simulink model "mdl"  (R2022b)
settings: Solver=VariableStepAuto  StartTime=0.0  StopTime=10.0  RelTol=1e-3
values from neighbouring files (symbols this model uses):
  acc_g = 9.8    [load_init_states.m]
  CG = [0;0;0]    [load_init_states.m]
  CP = [0;0;0]    [load_mdl_data.m]
  h0 = 1    [load_init_states.m]
  mass = 38    [load_init_states.m]
  maxP = 3000*0.8    (= 2400)    [load_mdl_data.m]
libraries: aerospace_common x3, aero x1, aerolibatmos2 x1
settings Model: Creator=matt  LastModifiedBy=matt
settings DataIOCC: ExternalInput=getinputstruct(spec1)  InitialState=getstatestruct(spec1)

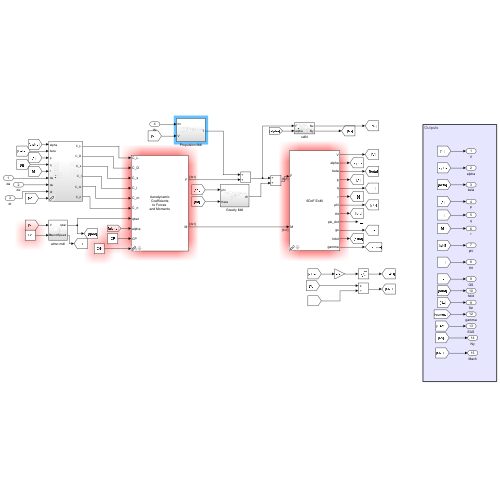
[thumbnail: Simulink's stored preview of the top-level diagram]
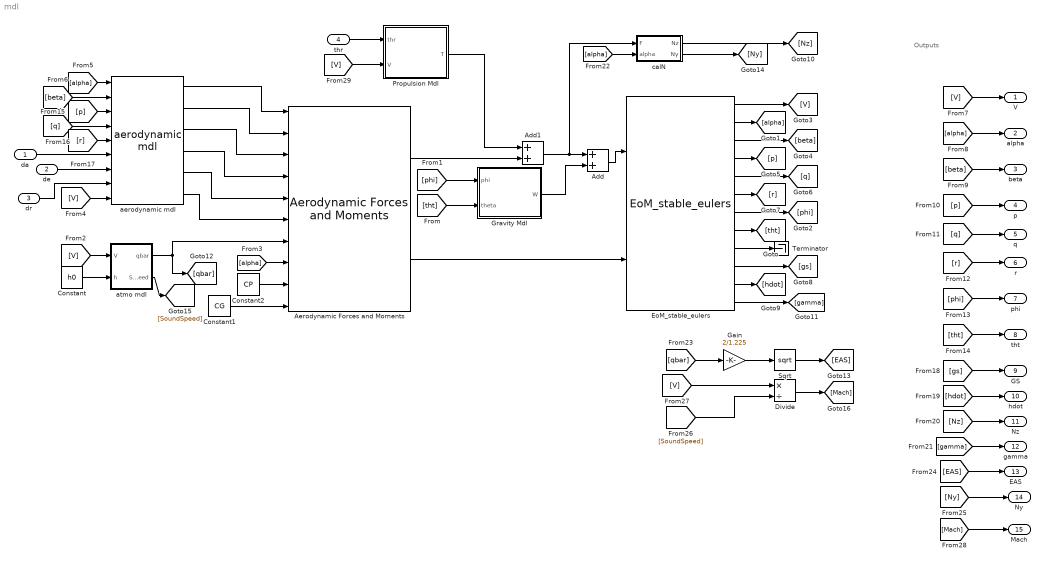
== system mdl ==
  note: Outputs
  da : Inport
  de : Inport  Port=2
  dr : Inport  Port=3
  thr : Inport  Port=4
  Add : Sum
  Add1 : Sum
  Aerodynamic Forces and Moments : aerospace_common/Aerodynamic Forces and Moments  RefArea=RefArea  RefLen=RefLen  RefSpan=RefSpan
  Constant : Constant  Value=h0
  Constant1 : Constant  Value=CG
  Constant2 : Constant  Value=CP
  Divide : Product  Inputs=*/
  EoM_stable_eulers : aerospace_common/EoM_stable_eulers  mass=mass  momentInertia=momentInertia  p0=0  q0=0  r0=0  V0=V0  alpha0=0.03  beta0=0  phi0=0  tht0=0  Parameter11=0
  Gain : Gain  Gain=2/1.225
  Gravity Mdl : Subsystem
  Propulsion Mdl : Subsystem
  Sqrt : Sqrt
  Terminator : Terminator
  aerodynamic mdl : aero/aerodynamic mdl  SystemSampleTime=-1  VariantActivationTime=update diagram  Latency=0  AutoFrameSizeCalculation=off
  atmo mdl : Subsystem
  calN : Subsystem
  V : Outport
  alpha : Outport  Port=2
  beta : Outport  Port=3
  p : Outport  Port=4
  q : Outport  Port=5
  r : Outport  Port=6
  phi : Outport  Port=7
  tht : Outport  Port=8
  GS : Outport  Port=9
  hdot : Outport  Port=10
  Nz : Outport  Port=11
  gamma : Outport  Port=12
  EAS : Outport  Port=13
  Ny : Outport  Port=14
  Mach : Outport  Port=15
  wires:
  Aerodynamic Forces and Moments/2 -> EoM_stable_eulers/2
  EoM_stable_eulers/1 -> [V]
  EoM_stable_eulers/2 -> [alpha]
  EoM_stable_eulers/3 -> [beta]
  EoM_stable_eulers/4 -> [p]
  EoM_stable_eulers/5 -> [q]
  EoM_stable_eulers/6 -> [r]
  EoM_stable_eulers/7 -> [phi]
  EoM_stable_eulers/8 -> [tht]
  EoM_stable_eulers/9 -> Terminator/1
  Aerodynamic Forces and Moments/1 -> Add1/2
  Add/1 -> EoM_stable_eulers/1
  Gravity Mdl/1(W) -> Add/2
  [tht] -> Gravity Mdl/2(theta)
  [phi] -> Gravity Mdl/1(phi)
  [V] -> atmo mdl/1(V)
  atmo mdl/1(qbar) -> Aerodynamic Forces and Moments/7, [qbar]
  Constant/1 -> atmo mdl/2(h)
  [alpha] -> Aerodynamic Forces and Moments/8
  aerodynamic mdl/1 -> Aerodynamic Forces and Moments/1
  aerodynamic mdl/2 -> Aerodynamic Forces and Moments/2
  aerodynamic mdl/3 -> Aerodynamic Forces and Moments/3
  aerodynamic mdl/4 -> Aerodynamic Forces and Moments/4
  aerodynamic mdl/5 -> Aerodynamic Forces and Moments/5
  aerodynamic mdl/6 -> Aerodynamic Forces and Moments/6
  da/1 -> aerodynamic mdl/6
  de/1 -> aerodynamic mdl/7
  dr/1 -> aerodynamic mdl/8
  [V] -> aerodynamic mdl/9
  [alpha] -> aerodynamic mdl/1
  [beta] -> aerodynamic mdl/2
  [V] -> V/1
  [alpha] -> alpha/1
  [beta] -> beta/1
  [p] -> p/1
  [q] -> q/1
  [r] -> r/1
  [phi] -> phi/1
  [tht] -> tht/1
  [p] -> aerodynamic mdl/3
  [q] -> aerodynamic mdl/4
  [r] -> aerodynamic mdl/5
  Propulsion Mdl/1(T) -> Add1/1
  thr/1 -> Propulsion Mdl/1(thr)
  EoM_stable_eulers/10 -> [gs]
  EoM_stable_eulers/11 -> [hdot]
  [gs] -> GS/1
  [hdot] -> hdot/1
  Add1/1 -> calN/1(F), Add/1
  EoM_stable_eulers/12 -> [gamma]
  calN/1(Nz) -> [Nz]
  [Nz] -> Nz/1
  [gamma] -> gamma/1
  Constant1/1 -> Aerodynamic Forces and Moments/10
  Constant2/1 -> Aerodynamic Forces and Moments/9
  [alpha] -> calN/2(alpha)
  [qbar] -> Gain/1
  Gain/1 -> Sqrt/1
  Sqrt/1 -> [EAS]
  [EAS] -> EAS/1
  calN/2(Ny) -> [Ny]
  [Ny] -> Ny/1
  atmo mdl/2(SoundSpeed) -> [SoundSpeed]
  [V] -> Divide/1
  [SoundSpeed] -> Divide/2
  Divide/1 -> [Mach]
  [Mach] -> Mach/1
  [V] -> Propulsion Mdl/2(V)

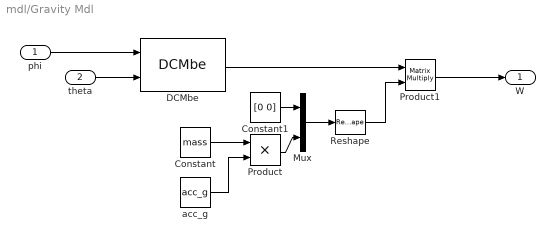
== system mdl/Gravity Mdl ==
  phi : Inport
  theta : Inport  Port=2
  Constant : Constant  Value=mass
  Constant1 : Constant  Value=[0 0]
  DCMbe : aerospace_common/DCMbe  SystemSampleTime=-1  VariantActivationTime=update diagram  Latency=0  AutoFrameSizeCalculation=off
      settings: LibrarySourceBlock=|
      | simulink/User-Defined
      | Functions/MATLAB Function
  Mux : Mux  Inputs=2
  Product : Product
  Product1 : Product  Multiplication=Matrix(*)
  Reshape : Reshape  OutputDimensionality=Column vector (2-D)
  acc_g : Constant  Value=acc_g
  W : Outport
  wires:
  Product1/1 -> W/1
  Product/1 -> Mux/2
  Constant1/1 -> Mux/1
  acc_g/1 -> Product/2
  Reshape/1 -> Product1/2
  Mux/1 -> Reshape/1
  Constant/1 -> Product/1
  DCMbe/1 -> Product1/1
  phi/1 -> DCMbe/1
  theta/1 -> DCMbe/2

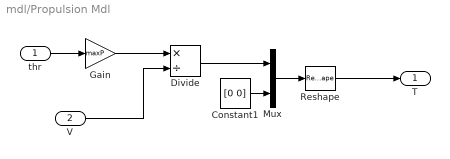
== system mdl/Propulsion Mdl ==
  thr : Inport
  V : Inport  Port=2
  Constant1 : Constant  Value=[0 0]
  Divide : Product  Inputs=*/
  Gain : Gain  Gain=maxP
  Mux : Mux  Inputs=2
  Reshape : Reshape  OutputDimensionality=Column vector (2-D)
  T : Outport
  wires:
  Reshape/1 -> T/1
  Mux/1 -> Reshape/1
  Constant1/1 -> Mux/2
  Divide/1 -> Mux/1
  thr/1 -> Gain/1
  Gain/1 -> Divide/1
  V/1 -> Divide/2

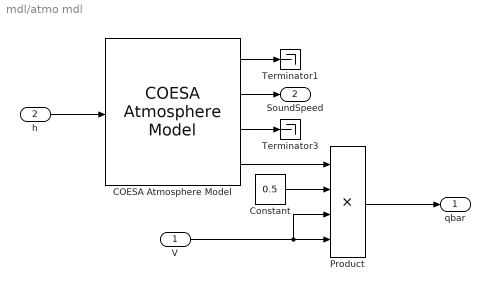
== system mdl/atmo mdl ==
  V : Inport
  h : Inport  Port=2
  COESA Atmosphere Model : aerolibatmos2/COESA Atmosphere Model  units=Metric (MKS)  spec=1976 COESA-extended U.S. Standard Atmosphere  model=Profile  profile_var=High temperature  profile_percent=1%  profile_alt=5 km (16404 ft)  envelope_var=High temperature  envelope_percent=1%  action=Warning
  Constant : Constant  Value=0.5
  Product : Product  Inputs=4
  Terminator1 : Terminator
  Terminator3 : Terminator
  qbar : Outport
  SoundSpeed : Outport  Port=2
  wires:
  COESA Atmosphere Model/2 -> SoundSpeed/1
  h/1 -> COESA Atmosphere Model/1
  COESA Atmosphere Model/3 -> Terminator3/1
  COESA Atmosphere Model/1 -> Terminator1/1
  COESA Atmosphere Model/4 -> Product/1
  Constant/1 -> Product/2
  V/1 -> Product/3, Product/4
  Product/1 -> qbar/1

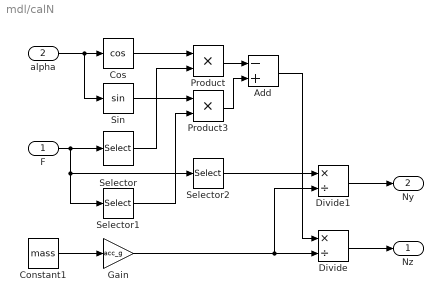
== system mdl/calN ==
  F : Inport
  alpha : Inport  Port=2
  Add : Sum  Inputs=-+
  Constant1 : Constant  Value=mass
  Cos : Trigonometry  Operator=cos
  Divide : Product  Inputs=*/
  Divide1 : Product  Inputs=*/
  Gain : Gain  Gain=acc_g
  Product : Product
  Product3 : Product
  Selector : Selector  IndexMode=Zero-based  InputPortWidth=3  IndexOptions=Index vector (dialog)  Indices=2  OutputSizes=1
  Selector1 : Selector  IndexMode=Zero-based  InputPortWidth=3  IndexOptions=Index vector (dialog)  Indices=0  OutputSizes=1
  Selector2 : Selector  IndexMode=Zero-based  InputPortWidth=3  IndexOptions=Index vector (dialog)  Indices=1  OutputSizes=1
  Sin : Trigonometry
  Nz : Outport
  Ny : Outport  Port=2
  wires:
  Gain/1 -> Divide1/2, Divide/2
  Constant1/1 -> Gain/1
  Divide/1 -> Nz/1
  F/1 -> Selector2/1, Selector1/1, Selector/1
  Selector/1 -> Product/2
  Add/1 -> Divide/1
  Cos/1 -> Product/1
  alpha/1 -> Sin/1, Cos/1
  Sin/1 -> Product3/1
  Selector1/1 -> Product3/2
  Product/1 -> Add/1
  Product3/1 -> Add/2
  Selector2/1 -> Divide1/1
  Divide1/1 -> Ny/1
